simulink model "regen"  (R2025b)
settings: Solver=VariableStepAuto  StartTime=0.0  StopTime=900  RelTol=1e-3
InitFcn:
  | speed_min = 6;
  | bpt_fmax = 60;
  | bpt_rmax = 60;
  | voltage_max = 299;
  | pedals_max = 0;
libraries: simulink x2
settings Model: Creator=benjaminlevin  LastModifiedBy=benjaminlevin

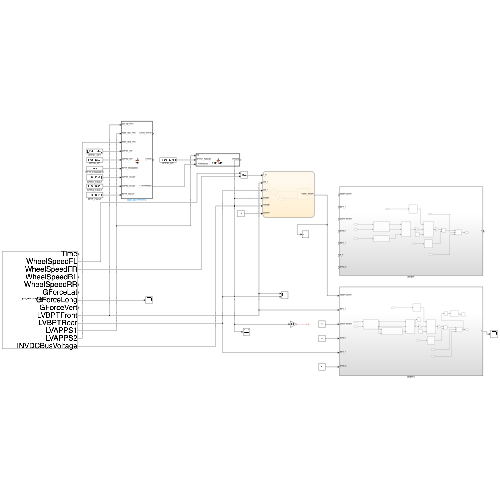
[thumbnail: Simulink's stored preview of the top-level diagram]
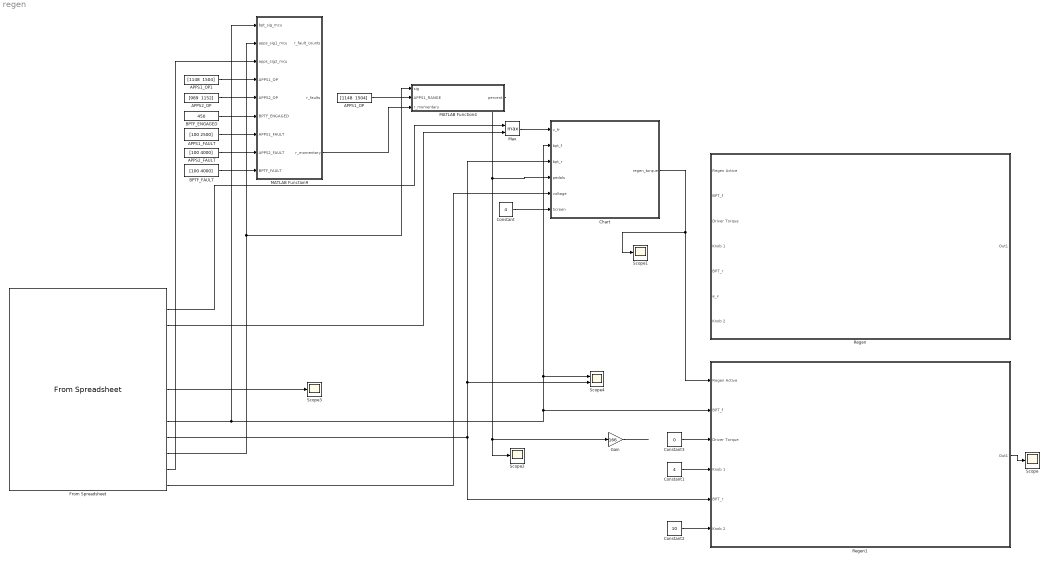
== system regen ==
  APPS1_FAULT : Constant  Value=[100 2500]  VectorParams1D=off
  APPS1_OP : Constant  Value="[1148  1504]"  VectorParams1D=off
  APPS1_OP1 : Constant  Value="[1148  1504]"  VectorParams1D=off
  APPS2_FAULT : Constant  Value=[100 4000]  VectorParams1D=off
  APPS2_OP : Constant  Value="[989  1152]"  VectorParams1D=off
  BPTF_ENGAGED : Constant  Value=450  VectorParams1D=off
  BPTF_FAULT : Constant  Value=[100 4000]  VectorParams1D=off
  Chart : Stateflow chart  TreatAsAtomicUnit=on
  Constant : Constant  Value=4
  Constant1 : Constant  Value=4
  Constant2 : Constant  Value=10
  Constant3 : Constant  Value=0
  From Spreadsheet : FromSpreadsheet  FileName=ryan_endurance_regen_test_long.xlsx  TreatFirstColumnAs=Data  SampleTime=0.002
  Gain : Gain  Gain=166
  MATLAB Function4 : MATLAB Function  TreatAsAtomicUnit=on
  MATLAB Function9 : MATLAB Function  TreatAsAtomicUnit=on
  Max : MinMax  Function=max  Inputs=2
  Regen : Subsystem
  Regen1 : Subsystem
  Scope{,1..3} (4 alike) : Scope
      Scope settings: ActiveDisplayYMinimum=-60.159801605657435  ActiveDisplayYMaximum=6.6844224006286019
      Scope1 settings: ActiveDisplayYMinimum=-0.12499999999999997  ActiveDisplayYMaximum=1.125
      Scope2 settings: ActiveDisplayYMinimum=-0.12499999999999997  ActiveDisplayYMaximum=1.125  DataLoggingVariableName=ScopeData3
      Scope3 settings: ActiveDisplayYMinimum=-1  ActiveDisplayYMaximum=1  DataLoggingVariableName=ScopeData4
  Scope4 : Scope  NumInputPorts=2
      settings: ActiveDisplayYMinimum=-97.374999999999972  ActiveDisplayYMaximum=866.375  DataLoggingVariableName=ScopeData5
  wires:
  Chart/1(regen_torque) -> Scope1/1, Regen1/1(Regen Active)
  MATLAB Function9/3(r_momentary) -> MATLAB Function4/3(r_momentary)
  APPS1_OP/1 -> MATLAB Function4/2(APPS1_RANGE)
  APPS1_OP1/1 -> MATLAB Function9/4(APPS1_OP)
  APPS2_OP/1 -> MATLAB Function9/5(APPS2_OP)
  BPTF_ENGAGED/1 -> MATLAB Function9/6(BPTF_ENGAGED)
  APPS1_FAULT/1 -> MATLAB Function9/7(APPS1_FAULT)
  APPS2_FAULT/1 -> MATLAB Function9/8(APPS2_FAULT)
  BPTF_FAULT/1 -> MATLAB Function9/9(BPTF_FAULT)
  Constant/1 -> Chart/6(Screen)
  Max/1 -> Chart/1(v_fr)
  MATLAB Function4/1(percent) -> Chart/4(pedals), Gain/1, Scope2/1
  Gain/1 -> ?
  Constant1/1 -> Regen1/4(Knob 1)
  Constant2/1 -> Regen1/6(Knob 2)
  From Spreadsheet/2 -> Max/1
  From Spreadsheet/3 -> Max/2
  From Spreadsheet/9 -> Chart/2(bpt_f), Scope4/1, Regen1/2(BPT_f), MATLAB Function9/1(bpt_sig_mcu)
  From Spreadsheet/10 -> Regen1/5(BPT_r), Chart/3(bpt_r), Scope4/2
  From Spreadsheet/11 -> MATLAB Function4/1(sig), MATLAB Function9/2(apps_sig1_mcu)
  From Spreadsheet/12 -> MATLAB Function9/3(apps_sig2_mcu)
  From Spreadsheet/13 -> Chart/5(voltage)
  Regen1/1(Out1) -> Scope/1
  From Spreadsheet/7 -> Scope3/1
  Constant3/1 -> Regen1/3(Driver Torque)

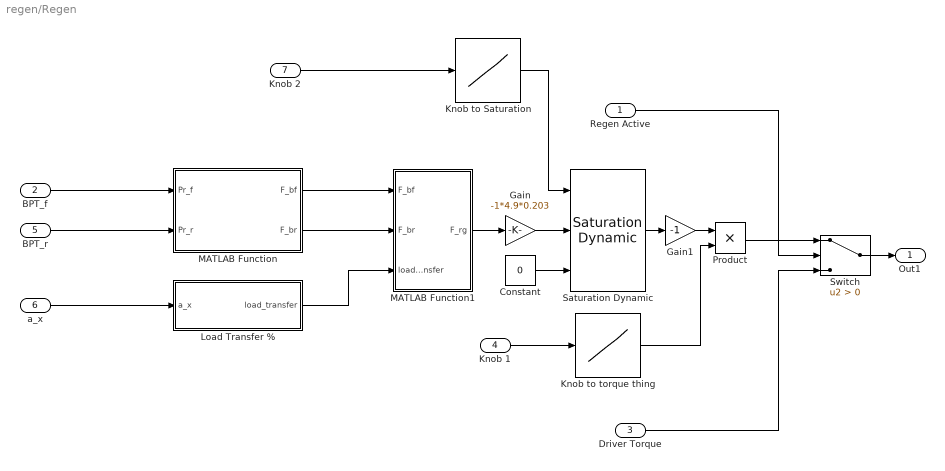
== system regen/Regen ==
  Regen Active : Inport
  BPT_f : Inport  Port=2
  Driver Torque : Inport  Port=3
  Knob 1 : Inport  Port=4
  BPT_r : Inport  Port=5
  a_x : Inport  Port=6
  Knob 2 : Inport  Port=7
  Constant : Constant  Value=0
  Gain : Gain  Gain=-1*4.9*0.203
  Gain1 : Gain  Gain=-1
  Knob to Saturation : Lookup_n-D  NumberOfTableDimensions=1  BreakpointsForDimension1=[1 10]  Table=[16.6 83]  InternalRulePriority=Speed  RndMeth=Simplest
  Knob to torque thing : Lookup_n-D  NumberOfTableDimensions=1  BreakpointsForDimension1=[1 10]  Table=[0 3]  InternalRulePriority=Speed  RndMeth=Simplest
  Load Transfer % : MATLAB Function  TreatAsAtomicUnit=on
  MATLAB Function : MATLAB Function  TreatAsAtomicUnit=on
  MATLAB Function1 : MATLAB Function  TreatAsAtomicUnit=on
  Product : Product
  Saturation Dynamic : simulink/Discontinuities/Saturation Dynamic  OutMin=[]  OutMax=[]  OutDataTypeStr=Inherit: Same as second input  OutDataType=fixdt(1, 16)  OutScaling=2^-10  DoSatur=off
  Switch : Switch  Criteria=u2 > Threshold  SaturateOnIntegerOverflow=off  InputSameDT=off
  Out1 : Outport
  wires:
  Switch/1 -> Out1/1
  Driver Torque/1 -> Switch/3
  Saturation Dynamic/1 -> Gain1/1
  Regen Active/1 -> Switch/2
  Knob to torque thing/1 -> Product/2
  Knob 1/1 -> Knob to torque thing/1
  BPT_f/1 -> MATLAB Function/1(Pr_f)
  BPT_r/1 -> MATLAB Function/2(Pr_r)
  a_x/1 -> Load Transfer %/1(a_x)
  MATLAB Function/1(F_bf) -> MATLAB Function1/1(F_bf)
  MATLAB Function/2(F_br) -> MATLAB Function1/2(F_br)
  Load Transfer %/1(load_transfer) -> MATLAB Function1/3(load_transfer)
  MATLAB Function1/1(F_rg) -> Gain/1
  Gain/1 -> Saturation Dynamic/2
  Gain1/1 -> Product/1
  Constant/1 -> Saturation Dynamic/3
  Knob 2/1 -> Knob to Saturation/1
  Knob to Saturation/1 -> Saturation Dynamic/1
  Product/1 -> Switch/1

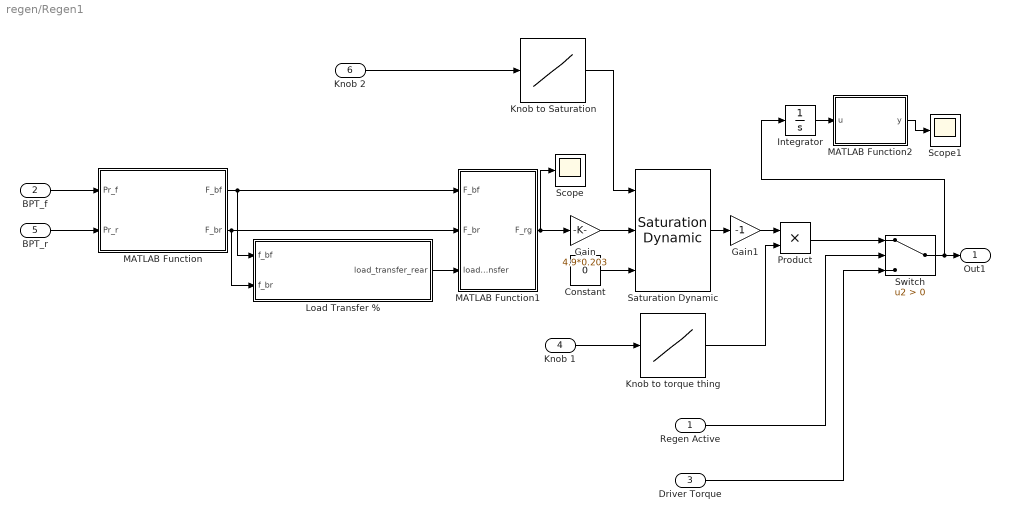
== system regen/Regen1 ==
  Regen Active : Inport
  BPT_f : Inport  Port=2
  Driver Torque : Inport  Port=3
  Knob 1 : Inport  Port=4
  BPT_r : Inport  Port=5
  Knob 2 : Inport  Port=6
  Constant : Constant  Value=0
  Gain : Gain  Gain=4.9*0.203
  Gain1 : Gain  Gain=-1
  Integrator : Integrator
  Knob to Saturation : Lookup_n-D  NumberOfTableDimensions=1  BreakpointsForDimension1=[1 10]  Table=[16.6 83]  InternalRulePriority=Speed  RndMeth=Simplest
  Knob to torque thing : Lookup_n-D  NumberOfTableDimensions=1  BreakpointsForDimension1=[1 10]  Table=[0 3]  InternalRulePriority=Speed  RndMeth=Simplest
  Load Transfer % : MATLAB Function  TreatAsAtomicUnit=on
  MATLAB Function : MATLAB Function  TreatAsAtomicUnit=on
  MATLAB Function1 : MATLAB Function  TreatAsAtomicUnit=on
  MATLAB Function2 : MATLAB Function  TreatAsAtomicUnit=on
  Product : Product
  Saturation Dynamic : simulink/Discontinuities/Saturation Dynamic  OutMin=[]  OutMax=[]  OutDataTypeStr=Inherit: Same as second input  OutDataType=fixdt(1, 16)  OutScaling=2^-10  DoSatur=off
  Scope : Scope
      settings: ActiveDisplayYMinimum=-1  ActiveDisplayYMaximum=1  DataLoggingVariableName=ScopeData2
  Scope1 : Scope
      settings: ActiveDisplayYMinimum=-162.22498582995041  ActiveDisplayYMaximum=18.024998425550042  DataLoggingVariableName=ScopeData6
  Switch : Switch  Criteria=u2 > Threshold  SaturateOnIntegerOverflow=off  InputSameDT=off
  Out1 : Outport
  wires:
  Switch/1 -> Integrator/1, Out1/1
  Driver Torque/1 -> Switch/3
  Saturation Dynamic/1 -> Gain1/1
  Regen Active/1 -> Switch/2
  Knob to torque thing/1 -> Product/2
  Knob 1/1 -> Knob to torque thing/1
  BPT_f/1 -> MATLAB Function/1(Pr_f)
  BPT_r/1 -> MATLAB Function/2(Pr_r)
  MATLAB Function/1(F_bf) -> MATLAB Function1/1(F_bf), Load Transfer %/1(f_bf)
  MATLAB Function/2(F_br) -> MATLAB Function1/2(F_br), Load Transfer %/2(f_br)
  Load Transfer %/1(load_transfer_rear) -> MATLAB Function1/3(load_transfer)
  Gain/1 -> Saturation Dynamic/2
  Gain1/1 -> Product/1
  Constant/1 -> Saturation Dynamic/3
  Knob 2/1 -> Knob to Saturation/1
  Knob to Saturation/1 -> Saturation Dynamic/1
  Product/1 -> Switch/1
  MATLAB Function1/1(F_rg) -> Gain/1, Scope/1
  Integrator/1 -> MATLAB Function2/1(u)
  MATLAB Function2/1(y) -> Scope1/1

== matlab function regen/Regen1/Load Transfer % ==
  data: f_bf input; load_transfer_rear output; f_br input
function load_transfer_rear = fcn(f_bf, f_br)
m = 250+68; %Mass with driver weight
a = 1.530/2; %Distance cg to front axle with load distribution of 0.5
h = 0.249; %Height of CG
l = 1.530; %Length of wheelbase
total_f = f_bf + f_br;
g = 9.81;
load_transfer_rear = abs((a*m*g)/l-(total_f*h)/l)/(m*g);

== matlab function regen/Regen1/MATLAB Function ==
  data: F_bf output; Pr_f input; F_br output; Pr_r input
function [F_bf,F_br] = fcn(Pr_f,Pr_r)
mu = 0.410;
r_rotor = 76.96; %mm, effective rotor radius
A_r = 1816; %mm^2
psi_to_bar = 1/14.503;
%maybe ((1/BB_e)-1), MIT paper, now is just some variable 0 to 1 minus 1
F_br = (2*mu*r_rotor*A_r*Pr_r*psi_to_bar)/(10000);
F_bf = (2*mu*r_rotor*A_r*Pr_f*psi_to_bar)/(10000);

== matlab function regen/Regen1/MATLAB Function1 ==
  data: F_rg output; F_bf input; F_br input; load_transfer input
function F_rg = fcn(F_bf,F_br,load_transfer)
F_rg = (F_bf+F_br)*load_transfer-F_br;

== matlab function regen/MATLAB Function4 ==
  data: sig input; APPS1_RANGE input; r_momentary input; percent output
function percent = map_apps1(sig, APPS1_RANGE, r_momentary)

DZ_BOT = .05; %rosnel changed to .05 was .1 
DZ_TOP = .05; 

APPS_BOTTOM = APPS1_RANGE(1) + DZ_BOT * (APPS1_RANGE(2) - APPS1_RANGE(1)) ;
APPS_TOP    = APPS1_RANGE(2) - DZ_TOP * (APPS1_RANGE(2) - APPS1_RANGE(1)) ;

if (sig < APPS_BOTTOM) || r_momentary(1) || r_momentary(2)
    percent = 0;
elseif sig > APPS_TOP
    percent = 1;
else
    percent = (double(sig) - APPS_BOTTOM) / (APPS_TOP - APPS_BOTTOM);
end

== matlab function regen/Regen1/MATLAB Function2 ==
  settings: updateMethod=DISCRETE
  data: u input; y output
function y = fcn(u)
persistent e;
if isempty(e)
    e = 0;
end
e = e + u;
y = e/(3600*1000);

== matlab function regen/MATLAB Function9 ==
  data: r_fault_counts output; r_faults output; bpt_sig_mcu input; apps_sig1_mcu input; apps_sig2_mcu input; APPS1_OP input; APPS2_OP input; BPTF_ENGAGED input; APPS1_FAULT input; APPS2_FAULT input; BPTF_FAULT input; r_momentary output
function [r_fault_counts, r_faults, r_momentary] = fcn(bpt_sig_mcu, apps_sig1_mcu, apps_sig2_mcu, APPS1_OP, APPS2_OP, BPTF_ENGAGED, APPS1_FAULT, APPS2_FAULT, BPTF_FAULT)
%#codegen
%To map voltages / integers:
%Pre step down voltages (from sensors, range 0 to 5 V) * 2/3 -> Post step down voltages (0 to 3.3 V, used by mcu)
%Post step down voltages * (4096 / 3.3) -> uint16 (integer) value of variables
%Note: Some values are tweaked after testing to handle noise. 455 -> 435, 0.1 -> 0.13, etc. All values can and should be optimized from testing, especially from testing on the car

%Current operating range (MCU): 0.32 V to 2.67 V
%Brakes considered pressed: 0.40 V
%typical MCU noise: +- 0.03V

persistent fault_counts;
persistent faults;

FAULT_LIMITS = [10, 10, 10, 10, 10, 10, 10, 1];

% initialize persistents
if isempty(fault_counts)
    fault_counts = zeros(1,8);
end

if isempty(faults)
    faults = [false, false, false, false, false, false, false, false];
end

apps1_percent_pressed = (double(apps_sig1_mcu) - APPS1_OP(1))/(APPS1_OP(2) - APPS1_OP(1)); % current travel divided by range of travel
apps2_percent_pressed = (double(apps_sig2_mcu) - APPS2_OP(1))/(APPS2_OP(2) - APPS2_OP(1));

% Clear fault case 8 (two pedals) when apps goes below 5% travel
if (apps1_percent_pressed < 0.05)
    faults(8) = 0;
    fault_counts(8) = 0;
end

% Cases 1-6: APPS or BPT out of operating range (sensor failure)
out_of_bounds = [apps_sig1_mcu < APPS1_FAULT(1), apps_sig1_mcu > APPS1_FAULT(2), ...
                 apps_sig2_mcu < APPS2_FAULT(1), apps_sig2_mcu > APPS2_FAULT(2), ...
                 bpt_sig_mcu   < BPTF_FAULT(1),  bpt_sig_mcu   > BPTF_FAULT(2)];
% Case 7: Both APPS sensors differ by more than 10% for more than 100ms. 
apps_disagree = abs(apps1_percent_pressed - apps2_percent_pressed) > 0.1;
% Case 8: If APPS is more than 25% pressed and brakes are pressed.
two_pedal = (apps1_percent_pressed >= 0.25) && (bpt_sig_mcu >= BPTF_ENGAGED);

conditions = [out_of_bounds, apps_disagree, two_pedal];

r_momentary = conditions;

conditions(8) = conditions(8) || faults(8); % Case 8 is sticky

% if condition is met but haven't yet triggered fault, increment fault_count.
% if condition is met but already in fault, leave fault_count the same (to
% prevent overflow)
% if condition is not met, zero the count
fault_counts = conditions .* (fault_counts + not(faults));
faults = fault_counts >= FAULT_LIMITS;

r_fault_counts = fault_counts;
r_faults = faults;

== matlab function regen/Regen/Load Transfer % ==
  data: a_x input; load_transfer output
function load_transfer = fcn(a_x)
m = 250+68; %Mass with driver weight
a = 1.530/2; %Distance cg to front axle with load distribution of 0.5
h = 0.249; %Height of CG
l = 1.530; %Length of wheelbase
load_transfer = abs(a_x*h/l);

== matlab function regen/Regen/MATLAB Function ==
  data: F_bf output; Pr_f input; F_br output; Pr_r input
function [F_bf,F_br] = fcn(Pr_f,Pr_r)
mu = 0.410;
r_rotor = 76.96; %mm, effective rotor radius
A_r = 1816; %mm^2
psi_to_bar = 1/14.503;
%maybe ((1/BB_e)-1), MIT paper, now is just some variable 0 to 1 minus 1
F_br = (2*mu*r_rotor*A_r*Pr_r*psi_to_bar)/(10000);
F_bf = (2*mu*r_rotor*A_r*Pr_f*psi_to_bar)/(10000);

== stateflow chart regen/Chart ==
  state REGEN_AVAILABLE
    regen_torque = 1;
  state REGEN_OFF
    regen_torque = 0;
  state REGEN_NOT_AVAILABLE
    regen_torque = 0;
  (default) -> REGEN_OFF
  REGEN_AVAILABLE -> REGEN_OFF [order 1] : [Screen <= 3]
  REGEN_NOT_AVAILABLE -> REGEN_OFF [order 1] : [Screen <= 3]
  REGEN_OFF -> REGEN_NOT_AVAILABLE : [Screen > 3]
  REGEN_NOT_AVAILABLE -> REGEN_AVAILABLE [order 2] : [v_fr > 0 & bpt_f > 5 & bpt_r > 5 & voltage < voltage_max & pedals <= pedals_max]
  REGEN_AVAILABLE -> REGEN_NOT_AVAILABLE [order 2] : [v_fr <= speed_min || bpt_f <= 5 || bpt_r <= 5 || voltage >= voltage_max || pedals > pedals_max]
  data: v_fr input; bpt_f input; bpt_r input; pedals input; voltage input; Screen input; regen_torque output double; pedals_max parameter; voltage_max parameter double; speed_min parameter

== matlab function regen/Regen/MATLAB Function1 ==
  data: F_rg output; F_bf input; F_br input; load_transfer input
function F_rg = fcn(F_bf,F_br,load_transfer)
gain = (0.5 - load_transfer)/(0.5+load_transfer);
F_rg = F_bf*gain-F_br;
